simulink model "mpc_ex_1"  (R2025b)
settings: Solver=VariableStepAuto  StartTime=0.0  StopTime=Tend  RelTol=1e-3
undefined symbols (not defined in the file): C, md
libraries: cstblocks x1
settings Model: Creator=davidecovolo  LastModifiedBy=davidecovolo

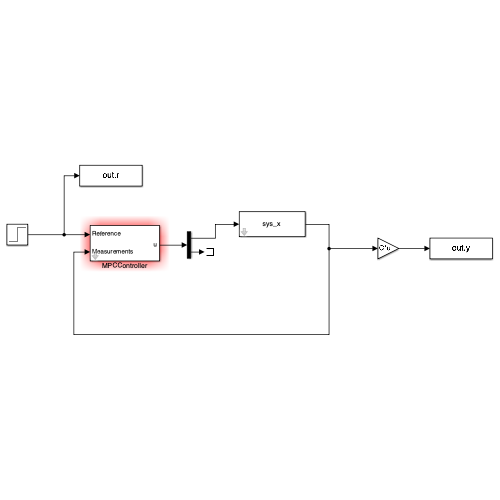
[thumbnail: Simulink's stored preview of the top-level diagram]
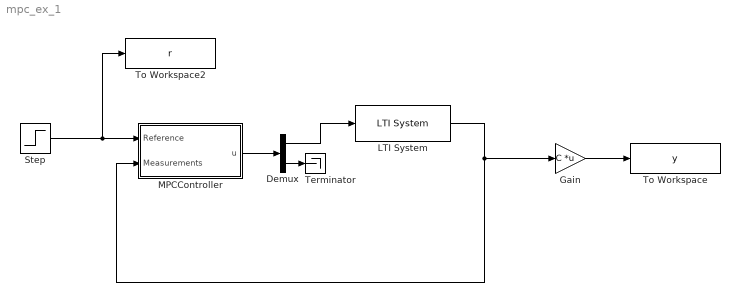
== system mpc_ex_1 ==
  Demux : Demux  Outputs=2
  Gain : Gain  Gain=C  Multiplication=Matrix(K*u)
  LTI System : cstblocks/LTI System  sys=sys_x  IC=[]  PadeOrder=0
  MPCController : Subsystem  mask{md=md}
      mask prompts: md "MPCData"
  Step : Step  Time=0  SampleTime=0
  Terminator : Terminator
  To Workspace : ToWorkspace  VariableName=y  SaveFormat=Timeseries  SampleTime=-1
  To Workspace2 : ToWorkspace  VariableName=r  SaveFormat=Timeseries  SampleTime=-1
  wires:
  Step/1 -> To Workspace2/1, MPCController/1(Reference)
  LTI System/1 -> MPCController/2(Measurements), Gain/1
  Gain/1 -> To Workspace/1
  MPCController/1(u) -> Demux/1
  Demux/1 -> LTI System/1
  Demux/2 -> Terminator/1

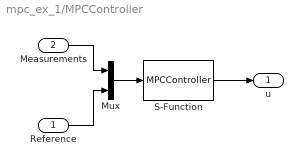
== system mpc_ex_1/MPCController ==
  Reference : Inport
  Measurements : Inport  Port=2
  Mux : Mux  Inputs=2
  S-Function : S-Function  FunctionName=MPCController  Parameters=md  SFunctionDeploymentMode=off  EnableBusSupport=off
  u : Outport
  wires:
  Mux/1 -> S-Function/1
  Measurements/1 -> Mux/1
  Reference/1 -> Mux/2
  S-Function/1 -> u/1
